simulink model "dfiir_df"  (R2023b)
settings: Solver=VariableStepAuto  StartTime=0.0  StopTime=10.0  RelTol=1e-3
undefined symbols (not defined in the file): a1, a2, b0, b1, b2
settings Model: Creator=eechris  LastModifiedBy=eechris

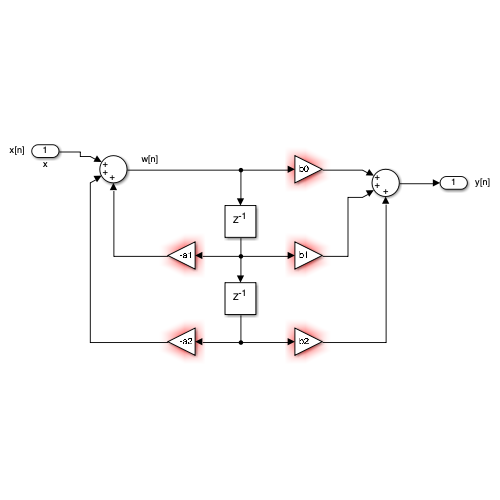
[thumbnail: Simulink's stored preview of the top-level diagram]
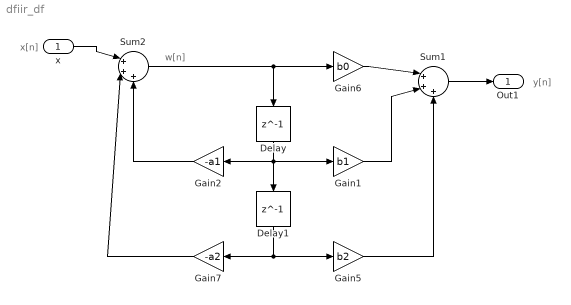
== system dfiir_df ==
  note: x[n]
  note: y[n]
  note: w[n]
  x : Inport
  Delay : Delay  DelayLength=1  InitialCondition=0
  Delay1 : Delay  DelayLength=1  InitialCondition=0
  Gain1 : Gain  Gain=b1
  Gain2 : Gain  Gain=-a1
  Gain5 : Gain  Gain=b2
  Gain6 : Gain  Gain=b0
  Gain7 : Gain  Gain=-a2
  Sum1 : Sum  Inputs=|+++
  Sum2 : Sum  Inputs=|+++
  Out1 : Outport
  wires:
  x/1 -> Sum2/1
  Gain2/1 -> Sum2/3
  Gain7/1 -> Sum2/2
  Delay/1 -> Gain1/1, Gain2/1, Delay1/1
  Sum2/1 -> Gain6/1, Delay/1
  Delay1/1 -> Gain7/1, Gain5/1
  Gain6/1 -> Sum1/1
  Gain1/1 -> Sum1/2
  Gain5/1 -> Sum1/3
  Sum1/1 -> Out1/1
